simulink model "wpr_hamsam"  (R2013a)
settings: Solver=ode4  StartTime=0.0  StopTime=5.0  FixedStep=0.001  RelTol=1e-3
values from neighbouring files (symbols this model uses):
  h = 40    [2.mat]    (also in 3.mat)
  k1 = 6000    [1.mat]    (also in 2.mat = 55000; 3.mat = 55000)
  k2 = 300000    [2.mat]    (also in 3.mat)
  m1 = 14000    [1.mat]    (also in 2.mat; 3.mat)
  m2 = 500    [2.mat]    (also in 3.mat)
  v0 = 70    [1.mat]    (also in 2.mat; 3.mat = 67)
settings Model: Creator=student  LastModifiedBy=adasdeb
settings DataIOCC: MaxDataPoints=10000  SignalLoggingSaveFormat=ModelDataLogs  TimeSaveName=toutwpr
settings OptimizationCC: ExpressionDepthLimit=2147483647
settings DebuggingCC: FcnCallInpInsideContextMsg=EnableAllAsWarning

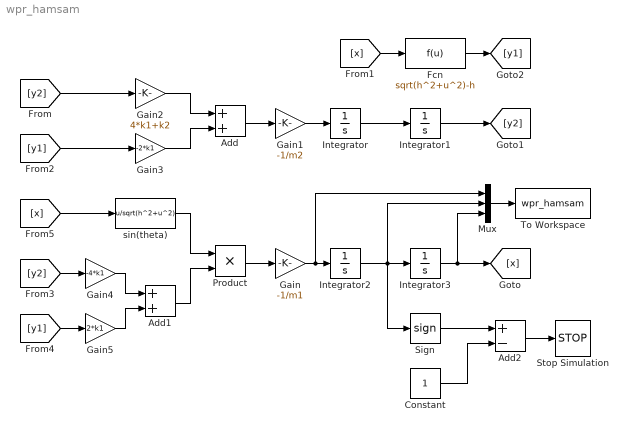
== system wpr_hamsam ==
  Add : Sum
  Add1 : Sum
  Add2 : Sum  Inputs=+-
  Constant : Constant
  Fcn : Fcn  Expr=sqrt(h^2+u^2)-h
  Gain : Gain  Gain=-1/m1
  Gain1 : Gain  Gain=-1/m2
  Gain2 : Gain  Gain=4*k1+k2
  Gain3 : Gain  Gain=-2*k1
  Gain4 : Gain  Gain=-4*k1
  Gain5 : Gain  Gain=2*k1
  Integrator : Integrator
  Integrator1 : Integrator
  Integrator2 : Integrator  InitialCondition=v0
  Integrator3 : Integrator
  Mux : Mux  Inputs=3
  Product : Product  RndMeth=Zero
  Sign : Signum
  Stop Simulation : Stop
  To Workspace : ToWorkspace  VariableName=wpr_hamsam  SampleTime=-1
  sin(theta) : Fcn  Expr=u/sqrt(h^2+u^2)
  wires:
  Integrator/1 -> Integrator1/1
  Gain1/1 -> Integrator/1
  Add/1 -> Gain1/1
  Gain/1 -> Mux/1, Integrator2/1
  Integrator3/1 -> Mux/3, [x]
  Integrator2/1 -> Mux/2, Sign/1, Integrator3/1
  Mux/1 -> To Workspace/1
  Integrator1/1 -> [y2]
  Sign/1 -> Add2/1
  Constant/1 -> Add2/2
  Add2/1 -> Stop Simulation/1
  [y2] -> Gain2/1
  Fcn/1 -> [y1]
  [x] -> Fcn/1
  [y1] -> Gain3/1
  Add1/1 -> Product/2
  sin(theta)/1 -> Product/1
  Product/1 -> Gain/1
  Gain5/1 -> Add1/2
  Gain4/1 -> Add1/1
  [y1] -> Gain5/1
  [y2] -> Gain4/1
  [x] -> sin(theta)/1
  Gain3/1 -> Add/2
  Gain2/1 -> Add/1
